simulink model "Two_DOF_SMsys"  (Simulink 9.3)
settings: Solver=VariableStepAuto  StartTime=0.0  StopTime=10.0  RelTol=1e-3
values from neighbouring files (symbols this model uses):
  c1 = 2.5    [MASS3.m]    (also in SMsysSIM.m = 2; three_MASS.m; two_DOF_sys_sim_ALL.m = 2)
  c2 = .5    (= 0.5)    [MASS3.m]    (also in SMsysSIM.m = 1; three_MASS.m; two_DOF_sys_sim_ALL.m = 1)
  c3 = 3.5    [MASS3.m]    (also in SMsysSIM.m = 3; three_MASS.m; two_DOF_sys_sim_ALL.m = 3)
  F0 = 3.3    [SMsysSIM.m]    (also in two_DOF_sys_sim_ALL.m)
  ICs = [theta1(0)==-.5,Dtheta1(0)==-1, theta2(0)==1, Dtheta2(0)==2]    [DOUBLE_Pedulum_Linear_2.m]    (also in LORENZ_functions.m = [-8, 8, 27]; Lotka_Voltera.m = [Alfa/Beta Gamma/Delta]; SMDsysSIM_compare.m = [0.1, 0]; SMsysSIM.m = [1; 1.5; -1; 1])
  k1 = 25    [MASS3.m]    (also in SMsysSIM.m = 90; three_MASS.m; two_DOF_sys_sim_ALL.m = 90)
  k2 = 5    [MASS3.m]    (also in SMsysSIM.m = 85; three_MASS.m; two_DOF_sys_sim_ALL.m = 85)
  m1 = 10    [DOUBLE_Pedulum_Linear_2.m]    (also in DOUBLE_Pedulum_Model_2.m; MASS3.m = 2.5; SMsysSIM.m = 5; three_MASS.m = 2.5)
  m2 = 10    [DOUBLE_Pedulum_Linear_2.m]    (also in DOUBLE_Pedulum_Model_2.m; MASS3.m = 2; SMsysSIM.m = 3; three_MASS.m = 2)
settings Model: Creator=sulaymon.eshkabilov  LastModifiedBy=sulaymon.eshkabilov
settings DataIOCC: SaveFormat=Dataset  SignalLoggingSaveFormat=Dataset  ReturnWorkspaceOutputs=on
settings OptimizationCC: LifeSpan=auto
settings DebuggingCC: UnderspecifiedInitializationDetection=Simplified  MergeDetectMultiDrivingBlocksExec=error  FcnCallInpInsideContextMsg=error  SFUnexpectedBacktrackingDiag=error  SFNoUnconditionalDefaultTransitionDiag=error  SFExecutionAtInitializationDiag=warning  ArithmeticOperatorsInVariantConditions=error
settings HardwareCC: ProdBitPerPointer=64  ProdBitPerSizeT=64  ProdBitPerPtrDiffT=64  ProdLargestAtomicFloat=Float  ProdIntDivRoundTo=Zero  ProdEndianess=LittleEndian  ProdWordSize=64  ProdHWDeviceType=Intel->x86-64 (Windows64)
settings ModelReferenceCC: PropagateSignalLabelsOutOfModel=on
settings SFSimCC: SimUseLocalCustomCode=on
settings RTWCC: RTWUseLocalCustomCode=on
settings CodeAppCC: StateflowObjectComments=off
settings GRTTargetCC: TargetLangStandard=C99 (ISO)  CombineOutputUpdateFcns=on  GRTInterface=off
settings ConfigComp: CovMetricSettings=dwe  CovHtmlReporting=off  CovSaveCumulativeToWorkspaceVar=off  CovSaveSingleToWorkspaceVar=off  CovExternalEMLEnable=on

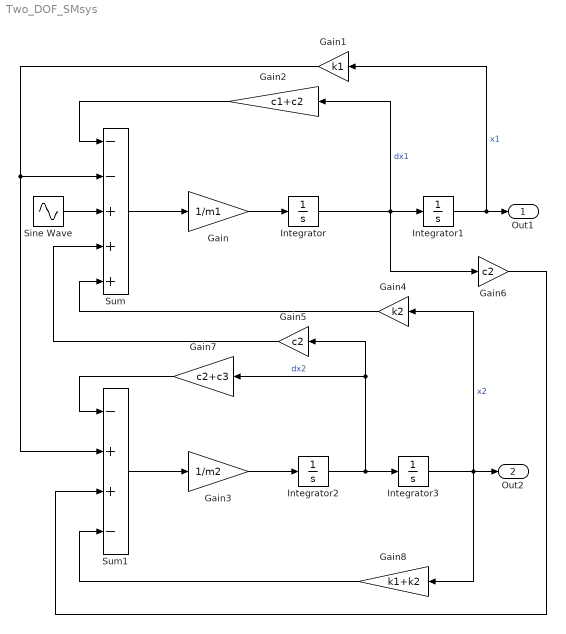
== system Two_DOF_SMsys ==
  Gain : Gain  Gain=1/m1
  Gain1 : Gain  Gain=k1
  Gain2 : Gain  Gain=c1+c2
  Gain3 : Gain  Gain=1/m2
  Gain4 : Gain  Gain=k2
  Gain5 : Gain  Gain=c2
  Gain6 : Gain  Gain=c2
  Gain7 : Gain  Gain=c2+c3
  Gain8 : Gain  Gain=k1+k2
  Integrator : Integrator  InitialCondition=ICs(2)
  Integrator1 : Integrator  InitialCondition=ICs(1)
  Integrator2 : Integrator  InitialCondition=ICs(4)
  Integrator3 : Integrator  InitialCondition=ICs(3)
  Sine Wave : Sin  Amplitude=F0  Frequency=10  SampleTime=0
  Sum : Sum  Inputs=--+++
  Sum1 : Sum  Inputs=-++-
  Out1 : Outport
  Out2 : Outport  Port=2
  wires:
  Sine Wave/1 -> Sum/3
  Gain/1 -> Integrator/1
  Integrator/1 -> Integrator1/1, Gain2/1, Gain6/1  "dx1"
  Integrator1/1 -> Out1/1, Gain1/1  "x1"
  Gain2/1 -> Sum/1
  Sum/1 -> Gain/1
  Gain3/1 -> Integrator2/1
  Integrator2/1 -> Integrator3/1, Gain5/1, Gain7/1  "dx2"
  Sum1/1 -> Gain3/1
  Gain5/1 -> Sum/4
  Gain4/1 -> Sum/5
  Integrator3/1 -> Out2/1, Gain8/1, Gain4/1  "x2"
  Gain7/1 -> Sum1/1
  Gain1/1 -> Sum1/2, Sum/2
  Gain8/1 -> Sum1/4
  Gain6/1 -> Sum1/3
